simulink model "prius_rulebased_2016"  (Simulink 8.7)
settings: Solver=ode4  SolverMode=SingleTasking  StartTime=0.0  StopTime=time_final  FixedStep=time_step  RelTol=1e-3  AbsTol=1e-6
values from neighbouring files (symbols this model uses):
  A_frontal = 2.52    [prius_sim_data.m]
  C_d = 0.3    [prius_sim_data.m]
  enable_stop = 1    [prius_sim_data.m]
  eng_consum_fuel = [0 0.654 0.328 0.238 0.232 0.257 0.29 0.323 0.353 0.381 0.407 0.435 0.465 0.501 0.545 0.599 0.665 0.746 0.842 0.957 ... (first row only)    [prius_sim_data.m]
  eng_ctrl_max_trq = [77.33 78.2 79.07 79.94 80.81 81.68 82.35 82.85 83.35 83.85              84.35 84.83 85.2 85.58 85.95 86.32 86.7 87.13 87.6 88.08 88.55              89.02 89.47 89.79 90.11 90.43 90.76 91.08 91.4 91.73 92.05 92.38              92.7 93.03 93.35 93.67 93.99 94.32 94.64 94.96 95.29 95.61 95.93              96.26 96.58 96.9 97.22 97.55 97.87 98.19 98.52 98.84 99.17 99.49              99.81 100.2 100.5 ...(+23 chars)    [prius_sim_init.m]
  eng_idle_spd = 1000*pi/30    (= 104.71975512)    [prius_sim_init.m]
  eng_pwr_max = 40000    [prius_sim_init.m]
  eng_pwr_opt = eng_spd_opt.*eng_ctrl_max_trq*0.9    [prius_sim_init.m]
  eng_spd_opt = eng_ctrl_spd    [prius_sim_init.m]
  ess_cap_scale = 1    [prius_sim_data.m]
  ess_fixtemp = 40    [prius_sim_data.m]
  ess_init_soc = soc_init_index(simrun)    [prius_sim_init.m]
  ess_max_ah_cap = [6.0 6.0]    [prius_sim_data.m]
  ess_max_volts = 9    [prius_sim_data.m]
  ess_min_volts = 6    [prius_sim_data.m]
  ess_module_num = 40    [prius_sim_data.m]
  ess_res_scale_coef = [1 0 1 0]    [prius_sim_data.m]
  ess_res_scale_fun = inline('(x(1)*ess_module_num+x(2))/(x(3)*ess_cap_scale+x(4))','x','ess_module_num','ess_cap_scale')    [prius_sim_data.m]
  ess_tmp = [0 25]    [prius_sim_data.m]
  f_rolling = 0.015    [prius_sim_data.m]
  FR = 3.905    [prius_sim_data.m]
  g_eff_map = 0.95*[ 0.88	0.89	0.90	0.91	0.90	0.79	0.79	0.79	0.90	0.91	0.90	0.89	0.88 ... (first row only)    [prius_sim_data.m]
  g_gravity = 9.81    [prius_sim_data.m]
  g_max_spd = [-200000 -10000 -8000 -6500 -5500 -4000 -3500 -3000 -2500 -2000 -1500 -1000 -500 0 500 1000 1500 2000 2500 3000 3500 4000 5500 6500 8000 10000 200000]*(2*pi)/60    [prius_sim_data.m]
  g_max_trq = 1.2*[0.01 14.3 18 22 26 36 41 48 55 55 55 55 55 55 55 55 55 55 55 48 41 36 26 22 18 14.3 0.01]    [prius_sim_data.m]
  gc_ki_on = 0.005    [prius_sim_init.m]
  gc_kp_on = 0.9    [prius_sim_init.m]
  gear_no = 4    [prius_sim_data.m]
  Kp_c = 30    [prius_sim_init.m]
  m_eff_map = 0.95*[ .905    .905    .905    .905    .905    .905    .905    .905    .905    .905    .905    .905	.905    .905    .905    .905    .905    .905    .905    .905    .905    .905    .905 ... (first row only)    [prius_sim_data.m]
  m_map_spd = [0 500 1000 1500 2000 2500 3000 3500 4000 4500  6000]*(2*pi)/60    [prius_sim_data.m]
  m_max_trq = interp1(m_spd_data,m_max_trq_data,m_map_spd,'linear')    [prius_sim_data.m]
  m_min_volts = 60    [prius_sim_data.m]
  M_total = 1.254*10^3    (= 1254)    [prius_sim_data.m]
  max_gen_spd = 6500*pi/30    (= 680.678408278)    [prius_sim_init.m]
  min_gen_spd = -6500*pi/30    (= -680.678408278)    [prius_sim_init.m]
  P_eng_mode = 40000    [prius_sim_init.m]
  P_ev_mode = 12000    [prius_sim_init.m]
  R_tire = 0.287    [prius_sim_data.m]
  regstop_soc = 0.8    [prius_sim_init.m]
  rho_air = 1.2    [prius_sim_data.m]
  soc_control = 0.55    [prius_sim_init.m]
  T2W = inv(W2T)    [prius_sim_data.m]
  target_soc = 0.6    [prius_sim_init.m]
  Ti_c = 60    [prius_sim_init.m]
  time_final = 1*length(cyc_mph(:,2))-1    [prius_sim_init.m]
  Tt_c = 65    [prius_sim_init.m]
  tx_pg_r = 78    [prius_sim_data.m]
  tx_pg_s = 30    [prius_sim_data.m]
  v_max_c = 100    [prius_sim_init.m]
  w_engine_on = 30*1600/3600/R_tire    [prius_sim_init.m]
undefined symbols (not defined in the file or in its folder): eng_map_trq
undefined symbols (not defined in the file): ess_r_chg, ess_r_dis, ess_soc, ess_voc
(part 2 of 2)

== system prius_rulebased_2016/Hybrid Controller/Drive/charging control ==
  soc : Inport
  Charging power limits : Inport  Port=2
  >0 : Saturate  UpperLimit=inf  LowerLimit=0
  Abs1 : Abs  SaturateOnIntegerOverflow=on
  Charging Controller Gain : Gain  Gain=1/0.1  SaturateOnIntegerOverflow=on  OutDataTypeStr=Inherit: Same as input  ParamDataTypeStr=Inherit: Same as input
  Constant1 : Constant  Value=15000
  Constant5 : Constant  Value=target_soc
  MinMax : MinMax  Inputs=2  SaturateOnIntegerOverflow=on  InputSameDT=on
  Product : Product  SaturateOnIntegerOverflow=on  OutDataTypeStr=Inherit: Same as first input
  Sum : Sum  Inputs=-+  SaturateOnIntegerOverflow=on
  Charging Power (W) : Outport
  wires:
  soc/1 -> Sum/1
  Charging power limits/1 -> Abs1/1  "Pch"
  Constant5/1 -> Sum/2
  Sum/1 -> Charging Controller Gain/1
  Charging Controller Gain/1 -> Product/2
  >0/1 -> Charging Power (W)/1
  MinMax/1 -> >0/1
  Product/1 -> MinMax/2
  Abs1/1 -> MinMax/1
  Constant1/1 -> Product/1

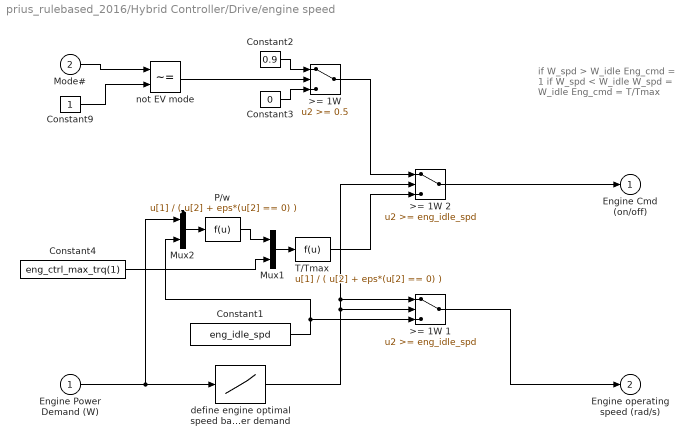
== system prius_rulebased_2016/Hybrid Controller/Drive/engine speed ==
  note: if W_spd > W_idle
      |   Eng_cmd = 1
      | if W_spd < W_idle
      |   W_spd = W_idle
      |   Eng_cmd = T/Tmax
  Engine Power Demand (W) : Inport
  Mode# : Inport  Port=2
  ">= 1W " : Switch  Threshold=0.5  SaturateOnIntegerOverflow=on  InputSameDT=on
  >= 1W 1 : Switch  Threshold=eng_idle_spd  SaturateOnIntegerOverflow=on  InputSameDT=on
  >= 1W 2 : Switch  Threshold=eng_idle_spd  SaturateOnIntegerOverflow=on  InputSameDT=on
  Constant1 : Constant  Value=eng_idle_spd
  Constant2 : Constant  Value=0.9
  Constant3 : Constant  Value=0
  Constant4 : Constant  Value=eng_ctrl_max_trq(1)
  Constant9 : Constant
  Mux1 : Mux  Inputs=2
  Mux2 : Mux  Inputs=2
  P/w : Fcn  Expr=u[1] / ( u[2] + eps*(u[2] == 0) )
  T/Tmax : Fcn  Expr=u[1] / ( u[2] + eps*(u[2] == 0) )
  define engine optimal speed base on power demand : Lookup  DialogController=Simulink.DDGSource  InputValues=eng_pwr_opt  Table=eng_spd_opt  SaturateOnIntegerOverflow=on
  not EV mode : RelationalOperator  Operator=~=  InputSameDT=on
  Engine Cmd (on/off) : Outport
  Engine operating speed (rad/s) : Outport  Port=2
  wires:
  Engine Power Demand (W)/1 -> define engine optimal speed base on power demand/1, Mux2/1
  Mode#/1 -> not EV mode/1
  Constant9/1 -> not EV mode/2
  not EV mode/1 -> ">= 1W "/2
  Constant2/1 -> ">= 1W "/1
  Constant3/1 -> ">= 1W "/3
  define engine optimal speed base on power demand/1 -> >= 1W 1/2, >= 1W 1/1, >= 1W 2/2
  Constant1/1 -> >= 1W 1/3, Mux2/2
  >= 1W 1/1 -> Engine operating speed (rad/s)/1
  Mux2/1 -> P/w/1
  ">= 1W "/1 -> >= 1W 2/1
  >= 1W 2/1 -> Engine Cmd (on/off)/1
  Mux1/1 -> T/Tmax/1
  P/w/1 -> Mux1/1
  Constant4/1 -> Mux1/2
  T/Tmax/1 -> >= 1W 2/3

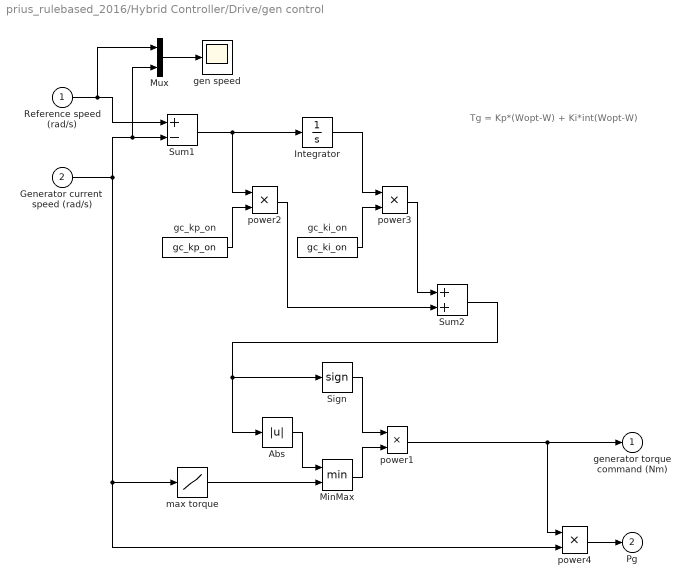
== system prius_rulebased_2016/Hybrid Controller/Drive/gen control ==
  note: Tg = Kp*(Wopt-W) + Ki*int(Wopt-W)
  Reference speed (rad/s) : Inport
  Generator current  speed (rad/s) : Inport  Port=2
  Abs : Abs  SaturateOnIntegerOverflow=on
  Integrator : Integrator
  MinMax : MinMax  Inputs=2  SaturateOnIntegerOverflow=on  InputSameDT=on
  Mux : Mux  Inputs=2
  Sign : Signum
  Sum1 : Sum  Inputs=+-  SaturateOnIntegerOverflow=on  InputSameDT=on  OutDataTypeStr=Inherit: Same as first input
  Sum2 : Sum  SaturateOnIntegerOverflow=on  InputSameDT=on  OutDataTypeStr=Inherit: Same as first input
  gc_ki_on : Constant  Value=gc_ki_on
  gc_kp_on : Constant  Value=gc_kp_on
  gen speed : Scope
  max torque : Lookup  DialogController=Simulink.DDGSource  InputValues=g_max_spd  Table=g_max_trq  SaturateOnIntegerOverflow=on
  power{1..4} (4 alike) : Product  SaturateOnIntegerOverflow=on  InputSameDT=on  OutDataTypeStr=Inherit: Same as first input
  generator torque command (Nm) : Outport
  Pg : Outport  Port=2
  wires:
  Abs/1 -> MinMax/1
  max torque/1 -> MinMax/2
  Sign/1 -> power1/1
  MinMax/1 -> power1/2
  Reference speed (rad/s)/1 -> Sum1/1, Mux/1
  Generator current  speed (rad/s)/1 -> Sum1/2, Mux/2, max torque/1, power4/2
  Sum1/1 -> power2/1, Integrator/1
  gc_kp_on/1 -> power2/2
  gc_ki_on/1 -> power3/2
  Integrator/1 -> power3/1
  power3/1 -> Sum2/1
  power2/1 -> Sum2/2
  Sum2/1 -> Sign/1, Abs/1
  Mux/1 -> gen speed/1
  power1/1 -> generator torque command (Nm)/1, power4/1
  power4/1 -> Pg/1

== system prius_rulebased_2016/Hybrid Controller/Drive/gen speed ==
  Target engine speed (rad/s) : Inport
  Ring Gear/Motor current speed (rad/s) : Inport  Port=2
  1+tx_pg_r/tx_pg_s : Gain  Gain=1+tx_pg_r/tx_pg_s  SaturateOnIntegerOverflow=on  OutDataTypeStr=Inherit: Same as input  ParamDataTypeStr=Inherit: Same as input
  Saturation min_gen,max_gen : Saturate  UpperLimit=max_gen_spd*0.9  LowerLimit=min_gen_spd*0.9
  Sum1 : Sum  Inputs=+-  SaturateOnIntegerOverflow=on  InputSameDT=on  OutDataTypeStr=Inherit: Same as first input
  tx_pg_r/tx_pg_s : Gain  Gain=tx_pg_r/tx_pg_s  SaturateOnIntegerOverflow=on  OutDataTypeStr=Inherit: Same as input  ParamDataTypeStr=Inherit: Same as input
  Reference generator speed (rad/s) : Outport
  wires:
  Saturation min_gen,max_gen/1 -> Reference generator speed (rad/s)/1
  tx_pg_r/tx_pg_s/1 -> Sum1/2
  1+tx_pg_r/tx_pg_s/1 -> Sum1/1
  Target engine speed (rad/s)/1 -> 1+tx_pg_r/tx_pg_s/1
  Ring Gear/Motor current speed (rad/s)/1 -> tx_pg_r/tx_pg_s/1
  Sum1/1 -> Saturation min_gen,max_gen/1

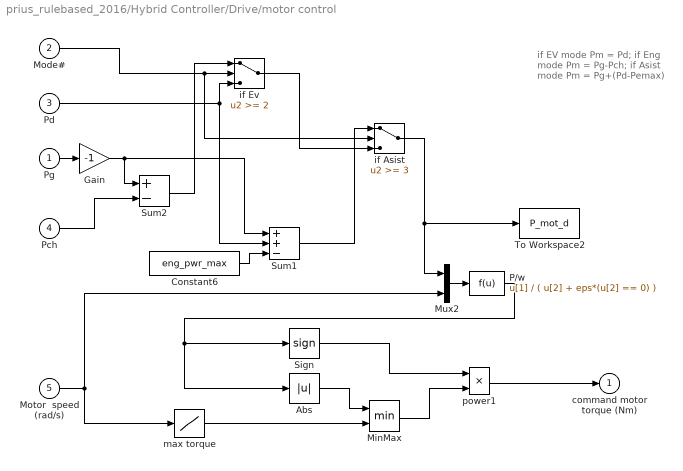
== system prius_rulebased_2016/Hybrid Controller/Drive/motor control ==
  note: if EV mode
      |    Pm = Pd;
      | if Eng mode
      |    Pm = Pg-Pch;
      | if Asist mode
      |    Pm = Pg+(Pd-Pemax)
  Pg : Inport
  Mode# : Inport  Port=2
  Pd : Inport  Port=3
  Pch : Inport  Port=4
  Motor  speed (rad/s) : Inport  Port=5
  Abs : Abs  SaturateOnIntegerOverflow=on
  Constant6 : Constant  Value=eng_pwr_max
  Gain : Gain  Gain=-1  SaturateOnIntegerOverflow=on  OutDataTypeStr=Inherit: Same as input  ParamDataTypeStr=Inherit: Same as input
  MinMax : MinMax  Inputs=2  SaturateOnIntegerOverflow=on  InputSameDT=on
  Mux2 : Mux  Inputs=2
  P/w : Fcn  Expr=u[1] / ( u[2] + eps*(u[2] == 0) )
  Sign : Signum
  Sum1 : Sum  Inputs=++-  SaturateOnIntegerOverflow=on  InputSameDT=on  OutDataTypeStr=Inherit: Same as first input
  Sum2 : Sum  Inputs=+-  SaturateOnIntegerOverflow=on  InputSameDT=on  OutDataTypeStr=Inherit: Same as first input
  To Workspace2 : ToWorkspace  VariableName=P_mot_d  SampleTime=-1
  if Asist : Switch  Threshold=3  SaturateOnIntegerOverflow=on  InputSameDT=on
  if Ev : Switch  Threshold=2  SaturateOnIntegerOverflow=on  InputSameDT=on
  max torque : Lookup  DialogController=Simulink.DDGSource  InputValues=m_map_spd  Table=m_max_trq  SaturateOnIntegerOverflow=on
  power1 : Product  SaturateOnIntegerOverflow=on  InputSameDT=on  OutDataTypeStr=Inherit: Same as first input
  command motor torque (Nm) : Outport  InitialOutput=0
  wires:
  Motor  speed (rad/s)/1 -> max torque/1, Mux2/2
  max torque/1 -> MinMax/2
  Mode#/1 -> if Ev/2, if Asist/2
  Pg/1 -> Gain/1
  Pch/1 -> Sum2/2
  Gain/1 -> Sum2/1, Sum1/1
  Sum2/1 -> if Ev/1
  Pd/1 -> if Ev/3, Sum1/2
  if Ev/1 -> if Asist/3
  Constant6/1 -> Sum1/3
  Sum1/1 -> if Asist/1
  Mux2/1 -> P/w/1
  if Asist/1 -> Mux2/1, To Workspace2/1
  P/w/1 -> Sign/1, Abs/1
  Abs/1 -> MinMax/1
  Sign/1 -> power1/1
  MinMax/1 -> power1/2
  power1/1 -> command motor torque (Nm)/1
